simulink model "BuckyWagon_01"  (Simulink 7.5)
settings: Solver=FixedStepDiscrete  StartTime=0.0  StopTime=10.0  RelTol=1e-3
PreLoadFcn:
  | try, eval([bdroot '_setup']); catch, eval('model_setup', ''); end
InitFcn:
  | try, eval([bdroot '_setup']); catch, eval('model_setup', ''); end
undefined symbols (not defined in the file): ECU565, High, Low, miniviewSetup, motohawk_build_version, motohawk_get_faults, motohawk_setup_toolchains, motohawk_trunc_name, motohawk_vardec_config_group, motohawk_vardec_path, tc, True
libraries: MotoHawk_lib x381, simulink x26, miniview_lib x10, motohawk_control_primitives_lib x8, motohawk_engine_lib x6, motohawk_annotations_lib x2
(part 4 of 6)

== system BuckyWagon_01/Strategy/Control Strategy/Reverse ==
  Inputs : Inport  OutDataType=sfix(16)  OutScaling=2^0
  Bus Selector2 : BusSelector  OutputSignals=Accel,VehicleSpeed,ReverseSw
  Chart : Stateflow chart  TreatAsAtomicUnit=on
  Constant : Constant  OutDataType=sfix(16)  OutScaling=2^0
  Switch : Switch  Criteria=u2 ~= 0
  motohawk_calibration : MotoHawk_lib/Calibration & Probing Blocks/motohawk_calibration  nam='fwdAccThres'  val=0.02  storage=Calibration  show_more=on  name_source=Use Parameter  data_type=Inherit from 'Default Value'  read_level=1  write_level=1  ovr_cals=on  view_as=Number  enum_struct={'Disabled', 'Enabled'}  vector_style=Wide Row  use_help_units=on  help='Accelerator must be below this to switch Rev->Fwd'  units='%'  use_header_enum=off  row_header_enum={}  col_header_enum={}  use_min_max=on  min_val=0  max_val=1  use_precision=off  precision=''  gain=1  offset=0  exp=1  use_mototune_group=off  mototune_group=motohawk_vardec_path(gcb)
  motohawk_calibration1 : MotoHawk_lib/Calibration & Probing Blocks/motohawk_calibration  nam='ReverseDerate'  val=-1  storage=Calibration  show_more=on  name_source=Use Parameter  data_type=Inherit from 'Default Value'  read_level=1  write_level=1  ovr_cals=on  view_as=Number  enum_struct={'Disabled', 'Enabled'}  vector_style=Wide Row  use_help_units=on  help='Torque Derating Factor in reverse'  units='%'  use_header_enum=off  row_header_enum={}  col_header_enum={}  use_min_max=on  min_val=-1  max_val=0  use_precision=off  precision=''  gain=1  offset=0  exp=1  use_mototune_group=off  mototune_group=motohawk_vardec_path(gcb)
  motohawk_calibration2 : MotoHawk_lib/Calibration & Probing Blocks/motohawk_calibration  nam='fwdSpdThres'  val=5  storage=Calibration  show_more=on  name_source=Use Parameter  data_type=Inherit from 'Default Value'  read_level=1  write_level=1  ovr_cals=on  view_as=Number  enum_struct={'Disabled', 'Enabled'}  vector_style=Wide Row  use_help_units=on  help='Must be below this speed to switch Rev->Fwd'  units='mph'  use_header_enum=off  row_header_enum={}  col_header_enum={}  use_min_max=on  min_val=0  max_val=inf  use_precision=off  precision=''  gain=1  offset=0  exp=1  use_mototune_group=off  mototune_group=motohawk_vardec_path(gcb)
  motohawk_calibration3 : MotoHawk_lib/Calibration & Probing Blocks/motohawk_calibration  nam='offTime'  val=20  storage=Calibration  show_more=on  name_source=Use Parameter  data_type=Inherit from 'Default Value'  read_level=1  write_level=1  ovr_cals=on  view_as=Number  enum_struct={'Disabled', 'Enabled'}  vector_style=Wide Row  use_help_units=on  help='Switch must be released this long to press again.'  units='%'  use_header_enum=off  row_header_enum={}  col_header_enum={}  use_min_max=on  min_val=0  max_val=inf  use_precision=on  precision='1.3'  gain=0.005  offset=0  exp=1  use_mototune_group=off  mototune_group=motohawk_vardec_path(gcb)
  motohawk_calibration4 : MotoHawk_lib/Calibration & Probing Blocks/motohawk_calibration  nam='revAccThres'  val=0.02  storage=Calibration  show_more=on  name_source=Use Parameter  data_type=Inherit from 'Default Value'  read_level=1  write_level=1  ovr_cals=on  view_as=Number  enum_struct={'Disabled', 'Enabled'}  vector_style=Wide Row  use_help_units=on  help='Accelerator must be below this to switch Fwd->Rev'  units='%'  use_header_enum=off  row_header_enum={}  col_header_enum={}  use_min_max=on  min_val=0  max_val=1  use_precision=off  precision=''  gain=1  offset=0  exp=1  use_mototune_group=off  mototune_group=motohawk_vardec_path(gcb)
  motohawk_calibration5 : MotoHawk_lib/Calibration & Probing Blocks/motohawk_calibration  nam='revSpdThres'  val=5  storage=Calibration  show_more=on  name_source=Use Parameter  data_type=Inherit from 'Default Value'  read_level=1  write_level=1  ovr_cals=on  view_as=Number  enum_struct={'Disabled', 'Enabled'}  vector_style=Wide Row  use_help_units=on  help='Must be below this speed to switch Fwd->Rev.'  units='mph'  use_header_enum=off  row_header_enum={}  col_header_enum={}  use_min_max=on  min_val=0  max_val=inf  use_precision=off  precision=''  gain=1  offset=0  exp=1  use_mototune_group=off  mototune_group=motohawk_vardec_path(gcb)
  motohawk_calibration6 : MotoHawk_lib/Calibration & Probing Blocks/motohawk_calibration  nam='onTime'  val=10  storage=Calibration  show_more=on  name_source=Use Parameter  data_type=Inherit from 'Default Value'  read_level=1  write_level=1  ovr_cals=on  view_as=Number  enum_struct={'Disabled', 'Enabled'}  vector_style=Wide Row  use_help_units=on  help='Switch must be pressed this long.'  units='%'  use_header_enum=off  row_header_enum={}  col_header_enum={}  use_min_max=on  min_val=0  max_val=inf  use_precision=on  precision='1.3'  gain=0.005  offset=0  exp=1  use_mototune_group=off  mototune_group=motohawk_vardec_path(gcb)
  motohawk_override_abs : MotoHawk_lib/Calibration & Probing Blocks/motohawk_override_abs  SystemSampleTime=-1  parent_name='In_Reverse'  parent_val=0  show_more=off  name_source=Use Parameter  parent_read_level=1  parent_override_level=1  view_as=Number  enum_struct={'Disabled', 'Enabled'}  use_help_units=off  parent_help=''  parent_units=''  use_min_max=off  parent_min=-inf  parent_max=inf  use_precision=off  parent_precision=''  parent_gain=1  parent_offset=0  parent_exp=1  use_mototune_group=off  parent_group=motohawk_vardec_path(gcb)
  motohawk_probe : MotoHawk_lib/Calibration & Probing Blocks/motohawk_probe  nam='In_Reverse'  show_more=off  name_source=Use Parameter  read_level=1  view_as=Number  enum_struct={'Disabled', 'Enabled'}  vector_style=Wide Row  use_help_units=off  help=''  units=''  use_header_enum=off  row_header_enum={}  col_header_enum={}  use_precision=off  precision=''  gain=1  offset=0  exp=1  use_mototune_group=off  mototune_group=motohawk_vardec_path(gcb)
  InReverse : Outport  OutDataType=sfix(16)  OutScaling=2^0
  ReverseMult : Outport  Port=2  OutDataType=sfix(16)  OutScaling=2^0
  wires:
  Inputs/1 -> Bus Selector2/1
  Chart/1(inReverse) -> motohawk_override_abs/1
  motohawk_override_abs/1 -> InReverse/1, motohawk_probe/1, Switch/2
  motohawk_calibration1/1 -> Switch/1
  Constant/1 -> Switch/3
  Switch/1 -> ReverseMult/1
  motohawk_calibration/1 -> Chart/4(fwdAccThres)
  motohawk_calibration2/1 -> Chart/5(fwdSpdThres)
  Bus Selector2/1 -> Chart/1(accel)  "<Accel>"
  Bus Selector2/2 -> Chart/2(speed)  "<VehicleSpeed>"
  Bus Selector2/3 -> Chart/3(revButton)  "<ReverseSw>"
  motohawk_calibration4/1 -> Chart/7(revAccThres)
  motohawk_calibration3/1 -> Chart/6(offTime)
  motohawk_calibration5/1 -> Chart/8(revSpdThres)
  motohawk_calibration6/1 -> Chart/9(onTime)

== system BuckyWagon_01/Strategy/MiniViewDisplay/Down Button ==
  CAN Receive Slot Trigger : MotoHawk_lib/CAN Blocks/CAN Receive Slot Trigger  Tag=Trigger  slot='miniview_button_down'  inherited=on  function_name=Trigger_CAN_Slot_miniview_button_down_1271p0004
  Demux : Demux  Outputs=2
  Subsystem : Subsystem
  Update : Outport  OutDataType=sfix(16)  OutScaling=2^0
  Down Asserted : Outport  Port=2  OutDataType=sfix(16)  OutScaling=2^0
  Down Count : Outport  Port=3  OutDataType=sfix(16)  OutScaling=2^0
  wires:
  Subsystem/2(Out2) -> Down Count/1
  Demux/2 -> Update/1
  CAN Receive Slot Trigger/1 -> Demux/1
  Demux/1 -> Subsystem/Trigger
  Subsystem/1(Out1) -> Down Asserted/1

== system BuckyWagon_01/Strategy/MiniViewDisplay/Enabled Subsystem ==
  In : Inport  OutDataType=sfix(16)  OutScaling=2^0
  Enable : EnablePort
  Out : Outport  OutDataType=sfix(16)  OutScaling=2^0
  wires:
  In/1 -> Out/1

== system BuckyWagon_01/Strategy/MiniViewDisplay/Enabled Subsystem1 ==
  In : Inport  OutDataType=sfix(16)  OutScaling=2^0
  Enable : EnablePort
  Out : Outport  OutDataType=sfix(16)  OutScaling=2^0
  wires:
  In/1 -> Out/1

== system BuckyWagon_01/Strategy/MiniViewDisplay/Enabled Subsystem2 ==
  In : Inport  OutDataType=sfix(16)  OutScaling=2^0
  Enable : EnablePort
  Out : Outport  OutDataType=sfix(16)  OutScaling=2^0
  wires:
  In/1 -> Out/1

== system BuckyWagon_01/Strategy/MiniViewDisplay/Function-Call Subsystem ==
  Value : Inport  OutDataType=sfix(16)  OutScaling=2^0
  function : TriggerPort  TriggerType=function-call
  motohawk_data_write : MotoHawk_lib/Data Storage Blocks/motohawk_data_write  source=Lookup By Name  structure=Scalar  operation=Write scalar into location by index  sz_vec=-1  sz_row=3  sz_col=2  typ=uint8  nam='listIndex'  checkNull=on  write_read_only=off  struct_inst_name='Struct1'  struct_name='MyStruct'
  wires:
  Value/1 -> motohawk_data_write/1

== system BuckyWagon_01/Strategy/MiniViewDisplay/Function-Call Subsystem1 ==
  Value : Inport  OutDataType=sfix(16)  OutScaling=2^0
  function : TriggerPort  TriggerType=function-call
  motohawk_data_write : MotoHawk_lib/Data Storage Blocks/motohawk_data_write  source=Lookup By Name  structure=Scalar  operation=Write scalar into location by index  sz_vec=-1  sz_row=3  sz_col=2  typ=uint8  nam='screen'  checkNull=on  write_read_only=off  struct_inst_name='Struct1'  struct_name='MyStruct'
  wires:
  Value/1 -> motohawk_data_write/1

== system BuckyWagon_01/Strategy/MiniViewDisplay/Function-Call Subsystem2 ==
  Value : Inport  OutDataType=sfix(16)  OutScaling=2^0
  function : TriggerPort  TriggerType=function-call
  motohawk_data_write : MotoHawk_lib/Data Storage Blocks/motohawk_data_write  source=Lookup By Name  structure=Scalar  operation=Write scalar into location by index  sz_vec=-1  sz_row=3  sz_col=2  typ=uint8  nam='singleIndex'  checkNull=on  write_read_only=off  struct_inst_name='Struct1'  struct_name='MyStruct'
  wires:
  Value/1 -> motohawk_data_write/1

== system BuckyWagon_01/Strategy/MiniViewDisplay/Function-Call Subsystem3 ==
  Value : Inport  OutDataType=sfix(16)  OutScaling=2^0
  function : TriggerPort  TriggerType=function-call
  motohawk_data_write : MotoHawk_lib/Data Storage Blocks/motohawk_data_write  source=Lookup By Name  structure=Vector  operation=Write entire data structure at once  sz_vec=2  sz_row=3  sz_col=2  typ=uint8  nam='dualIndex'  checkNull=on  write_read_only=off  struct_inst_name='Struct1'  struct_name='MyStruct'
  wires:
  Value/1 -> motohawk_data_write/1

== system BuckyWagon_01/Strategy/MiniViewDisplay/Function-Call Subsystem4 ==
  Value : Inport  OutDataType=sfix(16)  OutScaling=2^0
  function : TriggerPort  TriggerType=function-call
  motohawk_data_write : MotoHawk_lib/Data Storage Blocks/motohawk_data_write  source=Lookup By Name  structure=Vector  operation=Write entire data structure at once  sz_vec=4  sz_row=3  sz_col=2  typ=uint8  nam='quadIndex'  checkNull=on  write_read_only=off  struct_inst_name='Struct1'  struct_name='MyStruct'
  wires:
  Value/1 -> motohawk_data_write/1

== system BuckyWagon_01/Strategy/MiniViewDisplay/GetFaultName ==
  Chart : Stateflow chart  TreatAsAtomicUnit=on
  Fault Iterator : Subsystem  TreatAsAtomicUnit=on
  Unit Delay : UnitDelay  SampleTime=-1
  Unit Delay1 : UnitDelay  SampleTime=-1
  getStringLength : Stateflow chart  TreatAsAtomicUnit=on
  motohawk_calibration : MotoHawk_lib/Calibration & Probing Blocks/motohawk_calibration  nam='DisplayFaults'  val=1  storage=Calibration  show_more=on  name_source=Use Parameter  data_type=boolean  read_level=1  write_level=1  ovr_cals=on  view_as=Enumeration  enum_struct={'Disabled', 'Enabled'}  vector_style=Wide Row  use_help_units=on  help='Enable displaying faults when they are active.'  units=''  use_header_enum=off  row_header_enum={}  col_header_enum={}  use_min_max=off  min_val=-inf  max_val=inf  use_precision=off  precision=''  gain=1  offset=0  exp=1  use_mototune_group=off  mototune_group=motohawk_vardec_path(gcb)
  motohawk_calibration1 : MotoHawk_lib/Calibration & Probing Blocks/motohawk_calibration  nam='InvertMode'  val=0  storage=Calibration  show_more=on  name_source=Use Parameter  data_type=boolean  read_level=1  write_level=1  ovr_cals=on  view_as=Enumeration  enum_struct={'Normal', 'Inverted'}  vector_style=Wide Row  use_help_units=on  help='Sets the background color for the text.'  units=''  use_header_enum=off  row_header_enum={}  col_header_enum={}  use_min_max=off  min_val=-inf  max_val=inf  use_precision=off  precision=''  gain=1  offset=0  exp=1  use_mototune_group=off  mototune_group=motohawk_vardec_path(gcb)
  motohawk_calibration2 : MotoHawk_lib/Calibration & Probing Blocks/motohawk_calibration  nam='noErrText'  val=uint8([32 66 117 99 107 69 86 0 0 0])  storage=Calibration  show_more=on  name_source=Use Parameter  data_type=uint8  read_level=1  write_level=1  ovr_cals=on  view_as=Text  enum_struct={'Disabled', 'Enabled'}  vector_style=Wide Row  use_help_units=on  help='Text to display if there are no faults.'  units=''  use_header_enum=off  row_header_enum={}  col_header_enum={}  use_min_max=off  min_val=-inf  max_val=inf  use_precision=off  precision=''  gain=1  offset=0  exp=1  use_mototune_group=off  mototune_group=motohawk_vardec_path(gcb)
  motohawk_calibration3 : MotoHawk_lib/Calibration & Probing Blocks/motohawk_calibration  nam='dispLength'  val=6  storage=Calibration  show_more=on  name_source=Use Parameter  data_type=uint8  read_level=1  write_level=1  ovr_cals=on  view_as=Number  enum_struct={'Disabled', 'Enabled'}  vector_style=Wide Row  use_help_units=on  help='Number of characters to display when scrolling fault name.'  units=''  use_header_enum=off  row_header_enum={}  col_header_enum={}  use_min_max=on  min_val=0  max_val=9  use_precision=on  precision=''  gain=1  offset=0  exp=1  use_mototune_group=off  mototune_group=motohawk_vardec_path(gcb)
  motohawk_calibration4 : MotoHawk_lib/Calibration & Probing Blocks/motohawk_calibration  nam='lastScrollTime'  val=100  storage=Calibration  show_more=on  name_source=Use Parameter  data_type=uint16  read_level=1  write_level=1  ovr_cals=on  view_as=Number  enum_struct={'Disabled', 'Enabled'}  vector_style=Wide Row  use_help_units=on  help='Time to spend on the last view of the scroll'  units='s'  use_header_enum=off  row_header_enum={}  col_header_enum={}  use_min_max=on  min_val=0  max_val=5  use_precision=on  precision='1.3'  gain=0.005  offset=0  exp=1  use_mototune_group=off  mototune_group=motohawk_vardec_path(gcb)
  motohawk_calibration5 : MotoHawk_lib/Calibration & Probing Blocks/motohawk_calibration  nam='scrollTime'  val=40  storage=Calibration  show_more=on  name_source=Use Parameter  data_type=uint16  read_level=1  write_level=1  ovr_cals=on  view_as=Number  enum_struct={'Disabled', 'Enabled'}  vector_style=Wide Row  use_help_units=on  help='Time to spend on each view of the scroll'  units='s'  use_header_enum=off  row_header_enum={}  col_header_enum={}  use_min_max=on  min_val=0  max_val=5  use_precision=on  precision='1.3'  gain=0.005  offset=0  exp=1  use_mototune_group=off  mototune_group=motohawk_vardec_path(gcb)
  motohawk_calibration6 : MotoHawk_lib/Calibration & Probing Blocks/motohawk_calibration  nam='minTime'  val=300  storage=Calibration  show_more=on  name_source=Use Parameter  data_type=uint16  read_level=1  write_level=1  ovr_cals=on  view_as=Number  enum_struct={'Disabled', 'Enabled'}  vector_style=Wide Row  use_help_units=on  help='Minimum time to display each fault name.'  units='s'  use_header_enum=off  row_header_enum={}  col_header_enum={}  use_min_max=on  min_val=0  max_val=5  use_precision=on  precision='1.3'  gain=0.005  offset=0  exp=1  use_mototune_group=off  mototune_group=motohawk_vardec_path(gcb)
  motohawk_calibration7 : MotoHawk_lib/Calibration & Probing Blocks/motohawk_calibration  nam='firstScrollTime'  val=200  storage=Calibration  show_more=on  name_source=Use Parameter  data_type=uint16  read_level=1  write_level=1  ovr_cals=on  view_as=Number  enum_struct={'Disabled', 'Enabled'}  vector_style=Wide Row  use_help_units=on  help='Time to spend on first view of the scroll'  units='s'  use_header_enum=off  row_header_enum={}  col_header_enum={}  use_min_max=on  min_val=0  max_val=5  use_precision=on  precision='1.3'  gain=0.005  offset=0  exp=1  use_mototune_group=off  mototune_group=motohawk_vardec_path(gcb)
  motohawk_probe : MotoHawk_lib/Calibration & Probing Blocks/motohawk_probe  nam='minTimer'  show_more=on  name_source=Use Parameter  read_level=1  view_as=Number  enum_struct={'Disabled', 'Enabled'}  vector_style=Wide Row  use_help_units=off  help=''  units=''  use_header_enum=off  row_header_enum={}  col_header_enum={}  use_precision=on  precision='1.3'  gain=0.005  offset=0  exp=1  use_mototune_group=off  mototune_group=motohawk_vardec_path(gcb)
  motohawk_probe2 : MotoHawk_lib/Calibration & Probing Blocks/motohawk_probe  nam='scrollTimer'  show_more=on  name_source=Use Parameter  read_level=1  view_as=Number  enum_struct={'Disabled', 'Enabled'}  vector_style=Wide Row  use_help_units=off  help=''  units=''  use_header_enum=off  row_header_enum={}  col_header_enum={}  use_precision=on  precision='1.3'  gain=0.005  offset=0  exp=1  use_mototune_group=off  mototune_group=motohawk_vardec_path(gcb)
  motohawk_probe3 : MotoHawk_lib/Calibration & Probing Blocks/motohawk_probe  nam='scrollIndex'  show_more=off  name_source=Use Parameter  read_level=1  view_as=Number  enum_struct={'Disabled', 'Enabled'}  vector_style=Wide Row  use_help_units=off  help=''  units=''  use_header_enum=off  row_header_enum={}  col_header_enum={}  use_precision=off  precision=''  gain=1  offset=0  exp=1  use_mototune_group=off  mototune_group=motohawk_vardec_path(gcb)
  Name : Outport  OutDataType=sfix(16)  OutScaling=2^0
  Mode : Outport  Port=2  OutDataType=sfix(16)  OutScaling=2^0
  wires:
  Chart/6(getNewFault) -> Fault Iterator/Trigger
  Chart/2(text) -> Name/1
  Chart/1(mode) -> Mode/1
  Chart/3(minTimer) -> motohawk_probe/1
  Chart/4(scrollIndex) -> motohawk_probe3/1
  Chart/5(scrollTimer) -> motohawk_probe2/1
  motohawk_calibration/1 -> Chart/7(dispFaults)
  motohawk_calibration1/1 -> Chart/1(invertMode)
  motohawk_calibration2/1 -> Chart/2(noErrText)
  motohawk_calibration3/1 -> Chart/3(dispLength)
  Fault Iterator/2(valid) -> Unit Delay1/1
  Fault Iterator/1(Name) -> Unit Delay/1
  motohawk_calibration4/1 -> Chart/4(lastScrollTime)
  motohawk_calibration5/1 -> Chart/5(scrollTime)
  motohawk_calibration6/1 -> Chart/8(minTime)
  getStringLength/1(faultNameLength) -> Chart/9(faultNameLen)
  Unit Delay/1 -> Chart/10(faultName), getStringLength/1(faultName)
  Unit Delay1/1 -> Chart/11(faultValid)
  motohawk_calibration7/1 -> Chart/6(firstScrollTime)

== system BuckyWagon_01/Strategy/MiniViewDisplay/Menu Button ==
  CAN Receive Slot Trigger : MotoHawk_lib/CAN Blocks/CAN Receive Slot Trigger  Tag=Trigger  slot='miniview_button_menu'  inherited=on  function_name=Trigger_CAN_Slot_miniview_button_menu_1529p0004
  Demux : Demux  Outputs=2
  Subsystem : Subsystem
  Update : Outport  OutDataType=sfix(16)  OutScaling=2^0
  Menu Asserted : Outport  Port=2  OutDataType=sfix(16)  OutScaling=2^0
  Menu Count : Outport  Port=3  OutDataType=sfix(16)  OutScaling=2^0
  wires:
  Subsystem/1(Out1) -> Menu Asserted/1
  Demux/1 -> Subsystem/Trigger
  CAN Receive Slot Trigger/1 -> Demux/1
  Demux/2 -> Update/1
  Subsystem/2(Out2) -> Menu Count/1

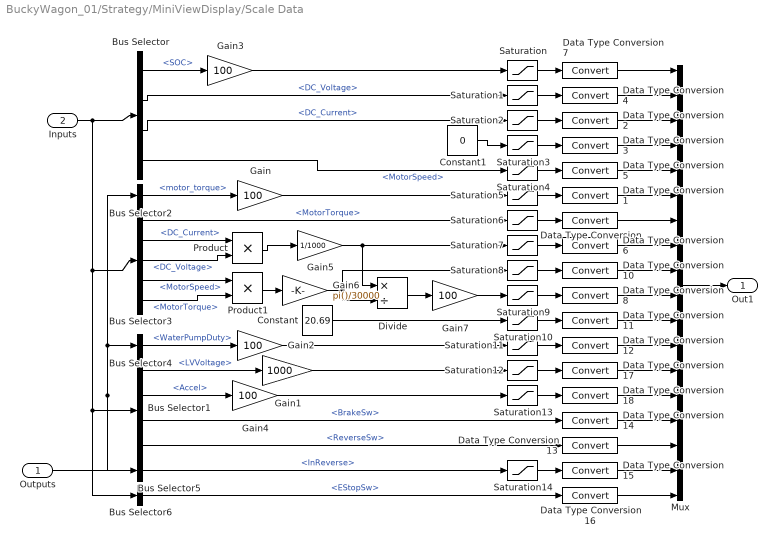
== system BuckyWagon_01/Strategy/MiniViewDisplay/Scale Data ==
  Outputs : Inport  OutDataType=sfix(16)  OutScaling=2^0
  Inputs : Inport  Port=2  OutDataType=sfix(16)  OutScaling=2^0
  Bus Selector : BusSelector  OutputSignals=SOC,DC_Voltage,DC_Current,MotorSpeed
  Bus Selector1 : BusSelector  OutputSignals=LVVoltage,Accel,BrakeSw,ReverseSw
  Bus Selector2 : BusSelector  OutputSignals=motor_torque
  Bus Selector3 : BusSelector  OutputSignals=MotorTorque,DC_Current,DC_Voltage,MotorSpeed,MotorTorque
  Bus Selector4 : BusSelector  OutputSignals=WaterPumpDuty
  Bus Selector5 : BusSelector  OutputSignals=InReverse
  Bus Selector6 : BusSelector  OutputSignals=EStopSw
  Constant : Constant  Value=20.69  OutDataType=fixdt(1, 16)  OutScaling=2^0
  Constant1 : Constant  Value=0  OutDataType=fixdt(1, 16)  OutScaling=2^0
  Data Type Conversion{,1..8,10..18} (18 alike) : DataTypeConversion  OutDataType=sfix(16)  OutScaling=2^0
  Divide : Product  Inputs=*/  OutDataType=sfix(16)  OutScaling=2^-10
  Gain{,2..4,7} (5 alike) : Gain  Gain=100  ParameterDataType=sfix(16)  ParameterScaling=2^0  OutDataType=sfix(16)  OutScaling=2^0  OutDataTypeStr=Inherit: Inherit via back propagation
  Gain1 : Gain  Gain=1000  ParameterDataType=sfix(16)  ParameterScaling=2^0  OutDataType=sfix(16)  OutScaling=2^0  OutDataTypeStr=Inherit: Inherit via back propagation
  Gain5 : Gain  Gain=1/1000  ParameterDataType=sfix(16)  ParameterScaling=2^0  OutDataType=sfix(16)  OutScaling=2^0  OutDataTypeStr=Inherit: Inherit via back propagation
  Gain6 : Gain  Gain=pi()/30000  ParameterDataType=sfix(16)  ParameterScaling=2^0  OutDataType=sfix(16)  OutScaling=2^0  OutDataTypeStr=Inherit: Inherit via back propagation
  Mux : Mux  Inputs=18
  Product : Product  OutDataType=sfix(16)  OutScaling=2^0  RndMeth=Zero
  Product1 : Product  OutDataType=sfix(16)  OutScaling=2^0  RndMeth=Zero
  Saturation{,1..8,10..14} (14 alike) : Saturate  UpperLimit=32767  LowerLimit=-32767  OutDataType=sfix(16)  OutScaling=2^0
  Saturation9 : Saturate  UpperLimit=100  LowerLimit=0  OutDataType=sfix(16)  OutScaling=2^0
  Out1 : Outport  OutDataType=sfix(16)  OutScaling=2^0
  wires:
  Outputs/1 -> Bus Selector2/1, Bus Selector4/1, Bus Selector5/1
  Bus Selector/3 -> Saturation2/1  "<DC_Current>"
  Bus Selector/2 -> Saturation1/1  "<DC_Voltage>"
  Bus Selector/1 -> Gain3/1  "<SOC>"
  Mux/1 -> Out1/1
  Gain3/1 -> Saturation/1
  Data Type Conversion4/1 -> Mux/2
  Data Type Conversion2/1 -> Mux/3
  Data Type Conversion3/1 -> Mux/4
  Data Type Conversion5/1 -> Mux/5
  Gain/1 -> Saturation5/1
  Bus Selector2/1 -> Gain/1  "<motor_torque>"
  Inputs/1 -> Bus Selector/1, Bus Selector3/1, Bus Selector1/1, Bus Selector6/1
  Bus Selector3/1 -> Saturation6/1  "<MotorTorque>"
  Bus Selector3/2 -> Product/1  "<DC_Current>"
  Bus Selector3/3 -> Product/2  "<DC_Voltage>"
  Product/1 -> Gain5/1
  Bus Selector3/4 -> Product1/1  "<MotorSpeed>"
  Bus Selector3/5 -> Product1/2  "<MotorTorque>"
  Product1/1 -> Gain6/1
  Constant/1 -> Saturation10/1
  Gain5/1 -> Divide/1, Saturation7/1
  Gain6/1 -> Divide/2, Saturation8/1
  Data Type Conversion/1 -> Mux/7
  Divide/1 -> Gain7/1
  Gain7/1 -> Saturation9/1
  Data Type Conversion6/1 -> Mux/8
  Data Type Conversion10/1 -> Mux/9
  Bus Selector4/1 -> Gain2/1  "<WaterPumpDuty>"
  Gain2/1 -> Saturation11/1
  Bus Selector1/1 -> Gain1/1  "<LVVoltage>"
  Bus Selector1/2 -> Gain4/1  "<Accel>"
  Bus Selector1/3 -> Data Type Conversion14/1  "<BrakeSw>"
  Bus Selector1/4 -> Data Type Conversion13/1  "<ReverseSw>"
  Gain1/1 -> Saturation12/1
  Gain4/1 -> Saturation13/1
  Data Type Conversion14/1 -> Mux/15
  Data Type Conversion13/1 -> Mux/16
  Bus Selector5/1 -> Saturation14/1  "<InReverse>"
  Data Type Conversion15/1 -> Mux/17
  Bus Selector6/1 -> Data Type Conversion16/1  "<EStopSw>"
  Data Type Conversion16/1 -> Mux/18
  Data Type Conversion1/1 -> Mux/6
  Data Type Conversion7/1 -> Mux/1
  Data Type Conversion8/1 -> Mux/10
  Data Type Conversion11/1 -> Mux/11
  Data Type Conversion12/1 -> Mux/12
  Data Type Conversion17/1 -> Mux/13
  Data Type Conversion18/1 -> Mux/14
  Saturation/1 -> Data Type Conversion7/1
  Saturation1/1 -> Data Type Conversion4/1
  Saturation2/1 -> Data Type Conversion2/1
  Saturation3/1 -> Data Type Conversion3/1
  Saturation4/1 -> Data Type Conversion5/1
  Saturation5/1 -> Data Type Conversion1/1
  Saturation6/1 -> Data Type Conversion/1
  Saturation7/1 -> Data Type Conversion6/1
  Saturation8/1 -> Data Type Conversion10/1
  Saturation9/1 -> Data Type Conversion8/1
  Saturation10/1 -> Data Type Conversion11/1
  Saturation11/1 -> Data Type Conversion12/1
  Saturation12/1 -> Data Type Conversion17/1
  Saturation13/1 -> Data Type Conversion18/1
  Saturation14/1 -> Data Type Conversion15/1
  Bus Selector/4 -> Saturation4/1  "<MotorSpeed>"
  Constant1/1 -> Saturation3/1

== system BuckyWagon_01/Strategy/MiniViewDisplay/Send String_efficient ==
  string # : Inport  OutDataType=sfix(16)  OutScaling=2^0
  string : Inport  Port=2  OutDataType=sfix(16)  OutScaling=2^0
  Trigger : TriggerPort  TriggerType=function-call
  Demux : Demux  Outputs=2
  Function-Call Generator : simulink/Ports & Subsystems/Function-Call Generator  sample_time=-1  numberOfIterations=1
  Signal Specification : SignalSpecification  Dimensions=18  DataType=uint8  OutDataType=sfix(16)  OutScaling=2^0  OutDataTypeStr=uint8
  Subsystem : Subsystem
  Next : Outport  OutDataType=sfix(16)  OutScaling=2^0
  wires:
  Signal Specification/1 -> Subsystem/2(string)
  Demux/2 -> Next/1
  Function-Call Generator/1 -> Demux/1
  Demux/1 -> Subsystem/Trigger
  string/1 -> Signal Specification/1  "b0"
  string #/1 -> Subsystem/1(string #)  "string"

== system BuckyWagon_01/Strategy/MiniViewDisplay/Up Button ==
  CAN Receive Slot Trigger : MotoHawk_lib/CAN Blocks/CAN Receive Slot Trigger  Tag=Trigger  slot='miniview_button_up'  inherited=on  function_name=Trigger_CAN_Slot_miniview_button_up_1778p0001
  Demux : Demux  Outputs=2
  Subsystem : Subsystem
  Update : Outport  OutDataType=sfix(16)  OutScaling=2^0
  Up Asserted : Outport  Port=2  OutDataType=sfix(16)  OutScaling=2^0
  Up Count : Outport  Port=3  OutDataType=sfix(16)  OutScaling=2^0
  wires:
  Subsystem/2(Up Count) -> Up Count/1
  Demux/2 -> Update/1
  CAN Receive Slot Trigger/1 -> Demux/1
  Demux/1 -> Subsystem/Trigger
  Subsystem/1(Up Asserted) -> Up Asserted/1

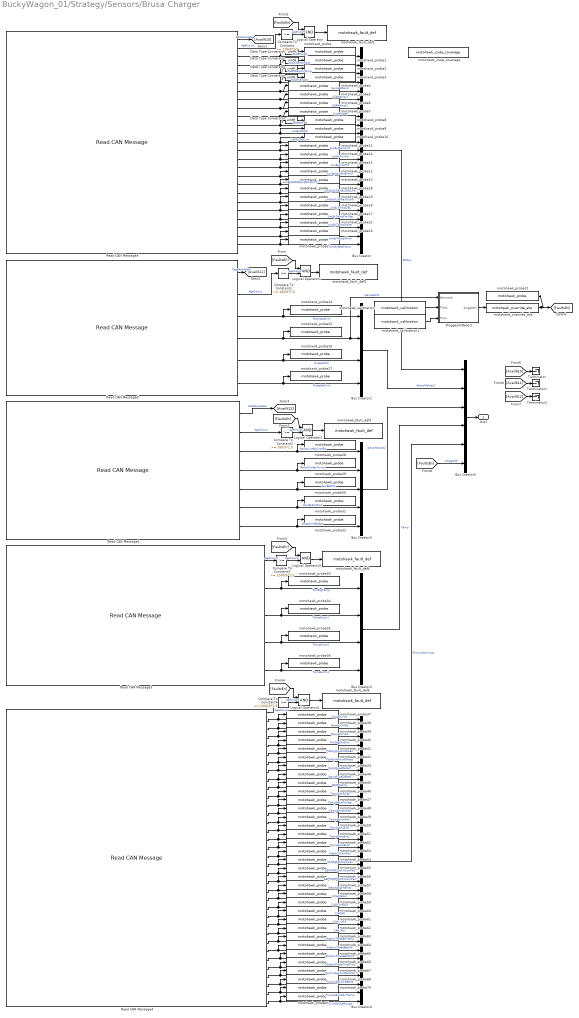
== system BuckyWagon_01/Strategy/Sensors/Brusa Charger ==
  Bus Creator : BusCreator  Inputs=23
  Bus Creator1 : BusCreator
  Bus Creator2 : BusCreator  Inputs=5
  Bus Creator3 : BusCreator
  Bus Creator4 : BusCreator  Inputs=34
  Bus Creator5 : BusCreator  Inputs=6
  Compare To Constant : simulink/Logic and Bit Operations/Compare To Constant  SystemSampleTime=-1  relop=>=  const=100/5*1.5  LogicOutDataTypeMode=boolean  ZeroCross=off
  Compare To Constant1 : simulink/Logic and Bit Operations/Compare To Constant  SystemSampleTime=-1  relop=>=  const=100/5*1.5  LogicOutDataTypeMode=boolean  ZeroCross=off
  Compare To Constant2 : simulink/Logic and Bit Operations/Compare To Constant  SystemSampleTime=-1  relop=>=  const=100/5*1.5  LogicOutDataTypeMode=boolean  ZeroCross=off
  Compare To Constant3 : simulink/Logic and Bit Operations/Compare To Constant  SystemSampleTime=-1  relop=>=  const=1000/5*1.5  LogicOutDataTypeMode=boolean  ZeroCross=off
  Compare To Constant4 : simulink/Logic and Bit Operations/Compare To Constant  SystemSampleTime=-1  relop=>=  const=1000/5*1.5  LogicOutDataTypeMode=boolean  ZeroCross=off
  Data Type Conversion{,1..4} (5 alike) : DataTypeConversion  OutDataTypeMode=uint8  OutDataType=sfix(16)  OutScaling=2^0  OutDataTypeStr=uint8
  Logical Operator{,1..4} (5 alike) : Logic  AllPortsSameDT=off  OutDataTypeMode=boolean  OutDataTypeStr=boolean
  PluggedInDetect : Subsystem
  Read CAN Message1 : MotoHawk_lib/CAN Blocks/Read CAN Message  nam=['CAN_' num2str(1)]  bus=-2  msg=can_BRUSA_612  queue=1  slot=''  valid=on  stale=on  labelwires=on
  Read CAN Message3 : MotoHawk_lib/CAN Blocks/Read CAN Message  nam=['CAN_' num2str(1)]  bus=-2  msg=can_BRUSA_613  queue=1  slot=''  valid=off  stale=on  labelwires=on
  Read CAN Message4 : MotoHawk_lib/CAN Blocks/Read CAN Message  nam=['CAN_' num2str(1)]  bus=-2  msg=can_BRUSA_614  queue=1  slot=''  valid=off  stale=on  labelwires=on
  Read CAN Message5 : MotoHawk_lib/CAN Blocks/Read CAN Message  nam=['CAN_' num2str(1)]  bus=-2  msg=can_BRUSA_610  queue=1  slot=''  valid=on  stale=on  labelwires=on
  Read CAN Message6 : MotoHawk_lib/CAN Blocks/Read CAN Message  nam=['CAN_' num2str(1)]  bus=-2  msg=can_BRUSA_611  queue=1  slot=''  valid=on  stale=on  labelwires=on
  Terminator : Terminator
  Terminator1 : Terminator
  Terminator2 : Terminator
  motohawk_calibration : MotoHawk_lib/Calibration & Probing Blocks/motohawk_calibration  nam='PluggedInMainsThes'  val=100  storage=Calibration  show_more=on  name_source=Use Parameter  data_type=Inherit from 'Default Value'  read_level=1  write_level=1  ovr_cals=on  view_as=Number  enum_struct={'Disabled', 'Enabled'}  vector_style=Wide Row  use_help_units=on  help='Above this mains voltage the charger is plugged in.'  units='V'  use_header_enum=off  row_header_enum={}  col_header_enum={}  use_min_max=off  min_val=-inf  max_val=inf  use_precision=off  precision=''  gain=1  offset=0  exp=1  use_mototune_group=off  mototune_group=motohawk_vardec_path(gcb)
  motohawk_calibration1 : MotoHawk_lib/Calibration & Probing Blocks/motohawk_calibration  nam='PluggedInHistTime'  val=300  storage=Calibration  show_more=on  name_source=Use Parameter  data_type=Inherit from 'Default Value'  read_level=1  write_level=1  ovr_cals=on  view_as=Number  enum_struct={'Disabled', 'Enabled'}  vector_style=Wide Row  use_help_units=on  help='Historesis time for plugged in detection.'  units='s'  use_header_enum=off  row_header_enum={}  col_header_enum={}  use_min_max=off  min_val=-inf  max_val=inf  use_precision=on  precision='1.2'  gain=0.005  offset=0  exp=1  use_mototune_group=off  mototune_group=motohawk_vardec_path(gcb)
  motohawk_code_coverage : MotoHawk_lib/Extra Development Blocks/motohawk_code_coverage
  motohawk_fault_def1 : MotoHawk_lib/Fault Management Blocks/motohawk_fault_def  nam='canNLG5_610'  mode=Disabled  id=0  x=10  y=40  input_suspected=on  indeterminate=off  increment_xy=on  downsample_count=1  ovr_cals=on  ovr_actions=off  show_actions=on  action1_name='Charge_Fault'  action1_cond=Active  action2_name=''  action2_cond=(None)  action3_name=''  action3_cond=(None)  action4_name=''  action4_cond=(None)
  motohawk_fault_def2 : MotoHawk_lib/Fault Management Blocks/motohawk_fault_def  nam='canNLG5_611'  mode=Disabled  id=0  x=10  y=40  input_suspected=on  indeterminate=off  increment_xy=on  downsample_count=1  ovr_cals=on  ovr_actions=off  show_actions=on  action1_name='Charge_Fault'  action1_cond=Active  action2_name=''  action2_cond=(None)  action3_name=''  action3_cond=(None)  action4_name=''  action4_cond=(None)
  motohawk_fault_def3 : MotoHawk_lib/Fault Management Blocks/motohawk_fault_def  nam='canNLG5_612'  mode=Disabled  id=0  x=10  y=40  input_suspected=on  indeterminate=off  increment_xy=on  downsample_count=1  ovr_cals=on  ovr_actions=off  show_actions=on  action1_name='Charge_Fault'  action1_cond=(None)  action2_name=''  action2_cond=(None)  action3_name=''  action3_cond=(None)  action4_name=''  action4_cond=(None)
  motohawk_fault_def4 : MotoHawk_lib/Fault Management Blocks/motohawk_fault_def  nam='canNLG5_613'  mode=Disabled  id=0  x=100  y=400  input_suspected=on  indeterminate=off  increment_xy=on  downsample_count=1  ovr_cals=on  ovr_actions=off  show_actions=off  action1_name=''  action1_cond=(None)  action2_name=''  action2_cond=(None)  action3_name=''  action3_cond=(None)  action4_name=''  action4_cond=(None)
  motohawk_fault_def5 : MotoHawk_lib/Fault Management Blocks/motohawk_fault_def  nam='canNLG5_614'  mode=Disabled  id=0  x=100  y=400  input_suspected=on  indeterminate=off  increment_xy=on  downsample_count=1  ovr_cals=on  ovr_actions=off  show_actions=off  action1_name=''  action1_cond=(None)  action2_name=''  action2_cond=(None)  action3_name=''  action3_cond=(None)  action4_name=''  action4_cond=(None)
  motohawk_override_abs : MotoHawk_lib/Calibration & Probing Blocks/motohawk_override_abs  SystemSampleTime=-1  parent_name='pluggedIn'  parent_val=0  show_more=off  name_source=Use Parameter  parent_read_level=1  parent_override_level=1  view_as=Number  enum_struct={'Disabled', 'Enabled'}  use_help_units=off  parent_help=''  parent_units=''  use_min_max=off  parent_min=-inf  parent_max=inf  use_precision=off  parent_precision=''  parent_gain=1  parent_offset=0  parent_exp=1  use_mototune_group=off  parent_group=motohawk_vardec_path(gcb)
  motohawk_probe : MotoHawk_lib/Calibration & Probing Blocks/motohawk_probe  nam='NLG5PwrEn'  show_more=on  name_source=Use Parameter  read_level=1  view_as=Enumeration  enum_struct={'Disabled', 'Enabled'}  vector_style=Wide Row  use_help_units=off  help=''  units=''  use_header_enum=off  row_header_enum={}  col_header_enum={}  use_precision=off  precision=''  gain=1  offset=0  exp=1  use_mototune_group=off  mototune_group=motohawk_vardec_path(gcb)
  motohawk_probe1 : MotoHawk_lib/Calibration & Probing Blocks/motohawk_probe  nam='NLG5GenErrLtch'  show_more=on  name_source=Use Parameter  read_level=1  view_as=Enumeration  enum_struct={'No Error', 'ERROR'}  vector_style=Wide Row  use_help_units=off  help=''  units=''  use_header_enum=off  row_header_enum={}  col_header_enum={}  use_precision=off  precision=''  gain=1  offset=0  exp=1  use_mototune_group=off  mototune_group=motohawk_vardec_path(gcb)
  motohawk_probe{4..7,9..20,22..70} (65 alike) : MotoHawk_lib/Calibration & Probing Blocks/motohawk_probe  nam='Probe'  show_more=on  name_source=Use Input Wire Name  read_level=1  view_as=Number  enum_struct={'Disabled', 'Enabled'}  vector_style=Wide Row  use_help_units=off  help=''  units=''  use_header_enum=off  row_header_enum={}  col_header_enum={}  use_precision=off  precision=''  gain=1  offset=0  exp=1  use_mototune_group=off  mototune_group=motohawk_vardec_path(gcb)
  motohawk_probe2 : MotoHawk_lib/Calibration & Probing Blocks/motohawk_probe  nam='NLG5GenLimWrng'  show_more=on  name_source=Use Parameter  read_level=1  view_as=Enumeration  enum_struct={'No Warn', 'WARNING'}  vector_style=Wide Row  use_help_units=off  help=''  units=''  use_header_enum=off  row_header_enum={}  col_header_enum={}  use_precision=off  precision=''  gain=1  offset=0  exp=1  use_mototune_group=off  mototune_group=motohawk_vardec_path(gcb)
  motohawk_probe21 : MotoHawk_lib/Calibration & Probing Blocks/motohawk_probe  nam='pluggedIn'  show_more=off  name_source=Use Parameter  read_level=1  view_as=Number  enum_struct={'Disabled', 'Enabled'}  vector_style=Wide Row  use_help_units=off  help=''  units=''  use_header_enum=off  row_header_enum={}  col_header_enum={}  use_precision=off  precision=''  gain=1  offset=0  exp=1  use_mototune_group=off  mototune_group=motohawk_vardec_path(gcb)
  motohawk_probe3 : MotoHawk_lib/Calibration & Probing Blocks/motohawk_probe  nam='NLG5FanActv'  show_more=on  name_source=Use Parameter  read_level=1  view_as=Enumeration  enum_struct={'Off', 'On'}  vector_style=Wide Row  use_help_units=off  help=''  units=''  use_header_enum=off  row_header_enum={}  col_header_enum={}  use_precision=off  precision=''  gain=1  offset=0  exp=1  use_mototune_group=off  mototune_group=motohawk_vardec_path(gcb)
  motohawk_probe8 : MotoHawk_lib/Calibration & Probing Blocks/motohawk_probe  nam='BypassDet'  show_more=on  name_source=Use Parameter  read_level=1  view_as=Enumeration  enum_struct={'none', 'DC', 'AC in Phase', 'AC not in Phase'}  vector_style=Wide Row  use_help_units=off  help=''  units=''  use_header_enum=off  row_header_enum={}  col_header_enum={}  use_precision=off  precision=''  gain=1  offset=0  exp=1  use_mototune_group=off  mototune_group=motohawk_vardec_path(gcb)
  Out1 : Outport  OutDataType=sfix(16)  OutScaling=2^0
  wires:
  Read CAN Message5/2 -> Compare To Constant/1  "AgeCount"
  Read CAN Message5/3 -> Bus Creator/1, Data Type Conversion/1  "NLG5PwrEn"
  Read CAN Message5/4 -> Bus Creator/2, Data Type Conversion1/1  "NLG5GenErrLtch"
  Read CAN Message5/5 -> Bus Creator/3, Data Type Conversion2/1  "NLG5GenLimWrng"
  Read CAN Message5/6 -> Bus Creator/4, Data Type Conversion3/1  "NLG5FanActv"
  Read CAN Message5/7 -> Bus Creator/5, motohawk_probe4/1  "EuropeMains"
  Read CAN Message5/8 -> Bus Creator/6, motohawk_probe5/1  "USAMainsL1"
  Read CAN Message5/9 -> Bus Creator/7, motohawk_probe6/1  "USAMainsL2"
  Read CAN Message5/10 -> Bus Creator/8, motohawk_probe7/1  "CntrlPltDet"
  Read CAN Message5/11 -> Bus Creator/9, Data Type Conversion4/1  "BypassDet"
  Read CAN Message5/12 -> Bus Creator/10, motohawk_probe9/1  "LimByOutVlt"
  Read CAN Message5/13 -> Bus Creator/11, motohawk_probe10/1  "LimByOutCrnt"
  Read CAN Message5/14 -> Bus Creator/12, motohawk_probe11/1  "LimByMainCrnt"
  Read CAN Message5/15 -> Bus Creator/13, motohawk_probe14/1  "LimByPwrInd"
  Read CAN Message5/16 -> Bus Creator/14, motohawk_probe15/1  "LimByCntrlPlt"
  Read CAN Message5/17 -> Bus Creator/15, motohawk_probe12/1  "LimByNLG5MaxPwr"
  Read CAN Message5/18 -> Bus Creator/16, motohawk_probe13/1  "LimByNLG5MaxMainsCrnt"
  Read CAN Message5/19 -> Bus Creator/17, motohawk_probe18/1  "LimByNLG5MaxOutCrnt"
  Read CAN Message5/20 -> Bus Creator/18, motohawk_probe19/1  "LimByNLG5MaxOutVlt"
  Read CAN Message5/21 -> Bus Creator/19, motohawk_probe16/1  "LimByTempCap"
  Read CAN Message5/22 -> Bus Creator/20, motohawk_probe17/1  "LimByTempPwrStg"
  Read CAN Message5/23 -> Bus Creator/21, motohawk_probe22/1  "LimByTempDiode"
  Read CAN Message5/24 -> Bus Creator/22, motohawk_probe23/1  "LimByTempXfrmr"
  Read CAN Message5/25 -> Bus Creator/23, motohawk_probe20/1  "LimByBattTemp"
  Read CAN Message1/3 -> motohawk_probe28/1, Bus Creator2/1  "MainsCrntByCntrlPlt"
  Read CAN Message1/4 -> motohawk_probe29/1, Bus Creator2/2  "MainsCrntByPwrInd"
  Read CAN Message1/5 -> motohawk_probe30/1, Bus Creator2/3  "AuxBattVlt"
  Read CAN Message1/6 -> motohawk_probe31/1, Bus Creator2/4  "AhrsByExtShnt"
  Read CAN Message1/7 -> Bus Creator2/5, motohawk_probe32/1  "OutptCrntByBstr"
  Read CAN Message1/2 -> Compare To Constant2/1  "AgeCount"
  Read CAN Message6/3 -> Bus Creator1/1, motohawk_probe24/1  "MainsActCrnt"
  Read CAN Message6/4 -> motohawk_probe25/1, Bus Creator1/2, PluggedInDetect/1(MainsVolt)  "MainsActVlt"
  Read CAN Message6/5 -> Bus Creator1/3, motohawk_probe26/1  "OutptActVlt"
  Read CAN Message6/6 -> Bus Creator1/4, motohawk_probe27/1  "OutptActCrnt"
  Read CAN Message3/1 -> Compare To Constant3/1  "AgeCount"
  Read CAN Message3/2 -> Bus Creator3/1, motohawk_probe33/1  "PwrStgTemp"
  Read CAN Message3/3 -> Bus Creator3/2, motohawk_probe34/1  "TempExtrn1"
  Read CAN Message3/4 -> Bus Creator3/3, motohawk_probe35/1  "TempExtrn2"
  Read CAN Message3/5 -> Bus Creator3/4, motohawk_probe36/1  "TempExtrn3"
  Read CAN Message4/1 -> Compare To Constant4/1  "AgeCount"
  Read CAN Message4/2 -> Bus Creator4/1, motohawk_probe37/1  "OutptOvrVlt"
  Read CAN Message4/3 -> Bus Creator4/2, motohawk_probe38/1  "MainsOvrVlt2"
  Read CAN Message4/4 -> Bus Creator4/3, motohawk_probe39/1  "MainsOvrVlt1"
  Read CAN Message4/5 -> Bus Creator4/4, motohawk_probe40/1  "PwrStgShrtCkt"
  Read CAN Message4/6 -> Bus Creator4/5, motohawk_probe41/1  "PlsbltyOutptVltMeas"
  Read CAN Message4/7 -> Bus Creator4/6, motohawk_probe42/1  "PlsbltyMainsVltMeas"
  Read CAN Message4/8 -> Bus Creator4/7, motohawk_probe43/1  "OutptFuseDefect"
  Read CAN Message4/9 -> Bus Creator4/8, motohawk_probe44/1  "MainsFuseDefect"
  Read CAN Message4/10 -> Bus Creator4/9, motohawk_probe45/1  "BattPolarity"
  Read CAN Message4/11 -> Bus Creator4/10, motohawk_probe46/1  "TempSensCap"
  Read CAN Message4/12 -> Bus Creator4/11, motohawk_probe47/1  "TempSensPwrStg"
  Read CAN Message4/13 -> Bus Creator4/12, motohawk_probe48/1  "TempSensDiode"
  Read CAN Message4/14 -> Bus Creator4/13, motohawk_probe49/1  "TempSensXfrmr"
  Read CAN Message4/15 -> Bus Creator4/14, motohawk_probe50/1  "TempSensExt1"
  Read CAN Message4/16 -> Bus Creator4/15, motohawk_probe51/1  "TempSensExt2"
  Read CAN Message4/17 -> Bus Creator4/16, motohawk_probe52/1  "TempSensExt3"
  Read CAN Message4/18 -> Bus Creator4/17, motohawk_probe53/1  "FlashChksmFail"
  Read CAN Message4/19 -> Bus Creator4/18, motohawk_probe54/1  "NVSRAMChksmFail"
  Read CAN Message4/20 -> Bus Creator4/19, motohawk_probe55/1  "EEPROMSysChksmFail"
  Read CAN Message4/21 -> Bus Creator4/20, motohawk_probe56/1  "EEPROMPOWChksmFail"
  Read CAN Message4/22 -> Bus Creator4/21, motohawk_probe57/1  "WatchdogInternal"
  Read CAN Message4/23 -> Bus Creator4/22, motohawk_probe58/1  "Initialization"
  Read CAN Message4/24 -> Bus Creator4/23, motohawk_probe59/1  "CANTimeout"
  Read CAN Message4/25 -> Bus Creator4/24, motohawk_probe60/1  "CANOff"
  Bus Creator/1 -> Bus Creator5/1  "Status"
  Bus Creator1/1 -> Bus Creator5/2  "ActualValues1"
  Bus Creator2/1 -> Bus Creator5/3  "ActualValues2"
  Bus Creator3/1 -> Bus Creator5/4  "Temp"
  Bus Creator4/1 -> Bus Creator5/5  "Errors/Warnings"
  Bus Creator5/1 -> Out1/1
  Read CAN Message4/26 -> Bus Creator4/25, motohawk_probe61/1  "CAN_Xmit"
  Read CAN Message4/27 -> Bus Creator4/26, motohawk_probe62/1  "CAN_Rcv"
  Read CAN Message4/28 -> Bus Creator4/27, motohawk_probe63/1  "ShtdwnThrsBattTemp"
  Read CAN Message4/29 -> Bus Creator4/28, motohawk_probe64/1  "ShtdwnThresBattVlt"
  Read CAN Message4/30 -> Bus Creator4/29, motohawk_probe65/1  "ShtdwnThresBattAhrs"
  Read CAN Message4/31 -> Bus Creator4/30, motohawk_probe66/1  "ShtdwnThresChrgTime"
  Read CAN Message4/32 -> Bus Creator4/31, motohawk_probe67/1  "PwrLimByLowMainsVlt"
  Read CAN Message4/33 -> Bus Creator4/32, motohawk_probe68/1  "PwrLimByLowBattVlt"
  Read CAN Message4/34 -> Bus Creator4/33, motohawk_probe70/1  "PwrLimByIntOvrTemp"
  Read CAN Message4/35 -> Bus Creator4/34, motohawk_probe69/1  "CmdValOutRange"
  Data Type Conversion/1 -> motohawk_probe/1
  Data Type Conversion1/1 -> motohawk_probe1/1
  Data Type Conversion2/1 -> motohawk_probe2/1
  Data Type Conversion3/1 -> motohawk_probe3/1
  Data Type Conversion4/1 -> motohawk_probe8/1
  [FaultsEn] -> Logical Operator/1
  Compare To Constant/1 -> Logical Operator/2  "AgeCount"
  Logical Operator/1 -> motohawk_fault_def1/1
  [FaultsEn] -> Logical Operator1/1
  Compare To Constant1/1 -> Logical Operator1/2  "AgeCount"
  Logical Operator1/1 -> motohawk_fault_def2/1
  [FaultsEn] -> Logical Operator2/1
  Compare To Constant2/1 -> Logical Operator2/2  "AgeCount"
  Logical Operator2/1 -> motohawk_fault_def3/1
  [FaultsEn] -> Logical Operator3/1
  Compare To Constant3/1 -> Logical Operator3/2  "AgeCount"
  Logical Operator3/1 -> motohawk_fault_def4/1
  [FaultsEn] -> Logical Operator4/1
  Compare To Constant4/1 -> Logical Operator4/2  "AgeCount"
  Logical Operator4/1 -> motohawk_fault_def5/1
  Read CAN Message5/1 -> [Avail610]  "DataAvailable"
  Read CAN Message6/2 -> Compare To Constant1/1  "AgeCount"
  Read CAN Message6/1 -> [Avail611]  "DataAvailable"
  Read CAN Message1/1 -> [Avail612]  "DataAvailable"
  [FaultsEn] -> Bus Creator5/6  "pluggedIn"
  motohawk_calibration/1 -> PluggedInDetect/2(Thres)
  motohawk_calibration1/1 -> PluggedInDetect/3(Time)
  PluggedInDetect/1(pluggedIn) -> motohawk_override_abs/1
  motohawk_override_abs/1 -> [FaultsEn], motohawk_probe21/1
  [Avail610] -> Terminator/1
  [Avail611] -> Terminator1/1
  [Avail612] -> Terminator2/1

== system BuckyWagon_01/Strategy/Sensors/EHPAS Power Steering Pump Inputts ==
  Compare To Constant3 : simulink/Logic and Bit Operations/Compare To Constant  SystemSampleTime=-1  relop=>  const=50/5*2  LogicOutDataTypeMode=boolean  ZeroCross=off
  Read CAN Message : MotoHawk_lib/CAN Blocks/Read CAN Message  nam='CAN_2'  bus=-2  msg=J1939_6A_PowerSteering_Status  queue=1  slot=''  valid=off  stale=on  labelwires=off
  Terminator5 : Terminator
  motohawk_fault_def3 : MotoHawk_lib/Fault Management Blocks/motohawk_fault_def  nam='PowerSteering_NoCAN_Status'  mode=Enabled  id=0  x=10  y=20  input_suspected=on  indeterminate=off  increment_xy=on  downsample_count=1  ovr_cals=on  ovr_actions=on  show_actions=off  action1_name=''  action1_cond=(None)  action2_name=''  action2_cond=(None)  action3_name=''  action3_cond=(None)  action4_name=''  action4_cond=(None)
  motohawk_probe{8..11,13..15} (7 alike) : MotoHawk_lib/Calibration & Probing Blocks/motohawk_probe  nam='Probe'  show_more=on  name_source=Use Input Wire Name  read_level=1  view_as=Number  enum_struct={'Disabled', 'Enabled'}  vector_style=Wide Row  use_help_units=off  help=''  units=''  use_header_enum=off  row_header_enum={}  col_header_enum={}  use_precision=off  precision=''  gain=1  offset=0  exp=1  use_mototune_group=on  mototune_group='Sensors | EHPAS'
  wires:
  Read CAN Message/1 -> Compare To Constant3/1  "AgeCount"
  Compare To Constant3/1 -> motohawk_fault_def3/1  "AgeCount"
  Read CAN Message/2 -> Terminator5/1
  Read CAN Message/3 -> motohawk_probe8/1  "EHPAS_Input_Voltage"
  Read CAN Message/4 -> motohawk_probe9/1  "EHPAS_Input_Current_NA"
  Read CAN Message/5 -> motohawk_probe10/1  "EHPAS_Pump_Speed"
  Read CAN Message/6 -> motohawk_probe11/1  "EHPAS_TempMax"
  Read CAN Message/7 -> motohawk_probe13/1  "EHPAS_TempCur"
  Read CAN Message/8 -> motohawk_probe14/1  "EHPAS_State"
  Read CAN Message/9 -> motohawk_probe15/1  "EHPAS_Fault"
